simulink model "testControlNavigation"  (R2021a)
settings: Solver=VariableStepAuto  StartTime=0.0  StopTime=200  RelTol=1e-3
values from neighbouring files (symbols this model uses):
  KK_PP = place(A, B, [s1, s2, s3, s4, s5, s6])    [control_extra3.m]
  Tmax = Fmax*Larm    (= 0.00125)    [control_extra3.m]
libraries: sharedtransform x2, simulink x1
settings Model: DataDictionary=databus.sldd  Creator=Laura  LastModifiedBy=Laura
settings SolverCC: ZeroCrossAlgorithm=Adaptive
settings DebuggingCC: MaskedZcDiagnostic=none  IgnoredZcDiagnostic=none

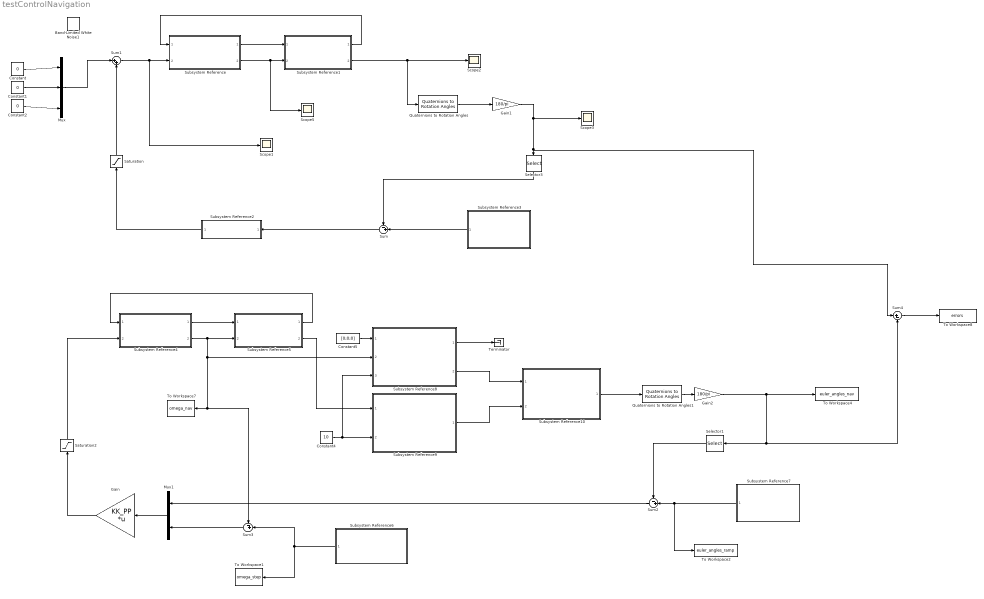
== system testControlNavigation ==
  Band-Limited White Noise1 : simulink/Sources/Band-Limited White Noise  Cov=[1e-11]  Ts=0.1  seed=[23341]
  Constant : Constant  Value=0
  Constant1 : Constant  Value=0
  Constant2 : Constant  Value=0
  Constant4 : Constant  Value=10
  Constant5 : Constant  Value=[0;0;0]
  Gain : Gain  Gain=KK_PP  Multiplication=Matrix(K*u)
  Gain1 : Gain  Gain=180/pi
  Gain2 : Gain  Gain=180/pi
  Mux : Mux  Inputs=3
  Mux1 : Mux  Inputs=2
  Quaternions to Rotation Angles : sharedtransform/Quaternions to Rotation Angles  rotationOrder=ZYX  aMode=aMode
      settings: SourceProductBaseCode=AE,PW,DR,MT,UV,VE
  Quaternions to Rotation Angles1 : sharedtransform/Quaternions to Rotation Angles  rotationOrder=ZYX  aMode=aMode
      settings: SourceProductBaseCode=AE,PW,DR,MT,UV,VE
  Saturation : Saturate  UpperLimit=Tmax  LowerLimit=-Tmax
  Saturation2 : Saturate  UpperLimit=Tmax  LowerLimit=-Tmax
  Scope{1..3,5} (4 alike) : Scope
  Selector1 : Selector  InputPortWidth=3  IndexOptions=Index vector (dialog)  Indices=[3 2 1]  OutputSizes=1
  Selector3 : Selector  InputPortWidth=3  IndexOptions=Index vector (dialog)  Indices=[3 2 1]  OutputSizes=1
  Subsystem Reference : Subsystem  ReferencedSubsystem=Dynamics
  Subsystem Reference1 : Subsystem  ReferencedSubsystem=Kinematics
  Subsystem Reference10 : Subsystem  ReferencedSubsystem=NavigationSolution
  Subsystem Reference2 : Subsystem  ReferencedSubsystem=PID
  Subsystem Reference3 : Subsystem  ReferencedSubsystem=ThreeAxesSignals
  Subsystem Reference4 : Subsystem  ReferencedSubsystem=Dynamics
  Subsystem Reference5 : Subsystem  ReferencedSubsystem=Kinematics
  Subsystem Reference6 : Subsystem  ReferencedSubsystem=AngVelocitySignals
  Subsystem Reference7 : Subsystem  ReferencedSubsystem=ThreeAxesSignals
  Subsystem Reference8 : Subsystem  ReferencedSubsystem=IMU
  Subsystem Reference9 : Subsystem  ReferencedSubsystem=StarTracker
  Sum : Sum  Inputs=-+|
  Sum1 : Sum  Inputs=|++
  Sum2 : Sum  Inputs=-+|
  Sum3 : Sum  Inputs=-+|
  Sum4 : Sum  Inputs=|+-
  Terminator : Terminator
  To Workspace1 : ToWorkspace  VariableName=omega_step  SaveFormat=Timeseries  SampleTime=-1
  To Workspace2 : ToWorkspace  VariableName=euler_angles_ramp  SaveFormat=Timeseries  SampleTime=-1
  To Workspace4 : ToWorkspace  VariableName=euler_angles_nav  SaveFormat=Timeseries  SampleTime=-1
  To Workspace7 : ToWorkspace  VariableName=omega_nav  SaveFormat=Timeseries  SampleTime=-1
  To Workspace8 : ToWorkspace  VariableName=errors  SaveFormat=Timeseries  SampleTime=-1
  wires:
  Subsystem Reference1/1 -> Subsystem Reference/1
  Subsystem Reference1/2 -> Scope2/1, Quaternions to Rotation Angles/1
  Subsystem Reference/2 -> Scope5/1, Subsystem Reference1/2
  Subsystem Reference/1 -> Subsystem Reference1/1
  Quaternions to Rotation Angles/1 -> Gain1/1
  Sum/1 -> Subsystem Reference2/1
  Subsystem Reference2/1 -> Saturation/1
  Selector3/1 -> Sum/1
  Sum1/1 -> Scope1/1, Subsystem Reference/2
  Saturation/1 -> Sum1/2
  Subsystem Reference3/1 -> Sum/2
  Gain2/1 -> Selector1/1, Sum4/2, To Workspace4/1
  Subsystem Reference7/1 -> To Workspace2/1, Sum2/2
  Sum2/1 -> Mux1/1
  Subsystem Reference4/1 -> Subsystem Reference5/1
  Quaternions to Rotation Angles1/1 -> Gain2/1
  Selector1/1 -> Sum2/1
  Subsystem Reference5/1 -> Subsystem Reference4/1
  Constant4/1 -> Subsystem Reference8/3, Subsystem Reference9/2
  Subsystem Reference5/2 -> Subsystem Reference9/1
  Constant5/1 -> Subsystem Reference8/1
  Subsystem Reference4/2 -> Sum3/1, To Workspace7/1, Subsystem Reference8/2, Subsystem Reference5/2
  Subsystem Reference8/1 -> Terminator/1
  Subsystem Reference9/1 -> Subsystem Reference10/2
  Subsystem Reference8/2 -> Subsystem Reference10/1
  Gain1/1 -> Scope3/1, Sum4/1, Selector3/1
  Sum4/1 -> To Workspace8/1
  Subsystem Reference10/1 -> Quaternions to Rotation Angles1/1
  Gain/1 -> Saturation2/1
  Mux/1 -> Sum1/1
  Constant/1 -> Mux/1
  Constant1/1 -> Mux/2
  Constant2/1 -> Mux/3
  Mux1/1 -> Gain/1
  Saturation2/1 -> Subsystem Reference4/2
  Sum3/1 -> Mux1/2
  Subsystem Reference6/1 -> To Workspace1/1, Sum3/2
